simulink subsystem "Funcionamiento_motores"  (R2023b)
settings: Solver=VariableStepAuto  StartTime=0.0  StopTime=10.0  RelTol=1e-3
libraries: arduinolib x4
settings Model: Creator=Usuario_UMA  LastModifiedBy=juana

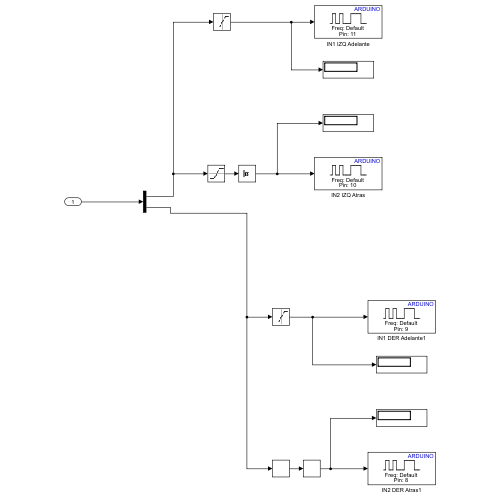
[thumbnail: Simulink's stored preview of the top-level diagram]
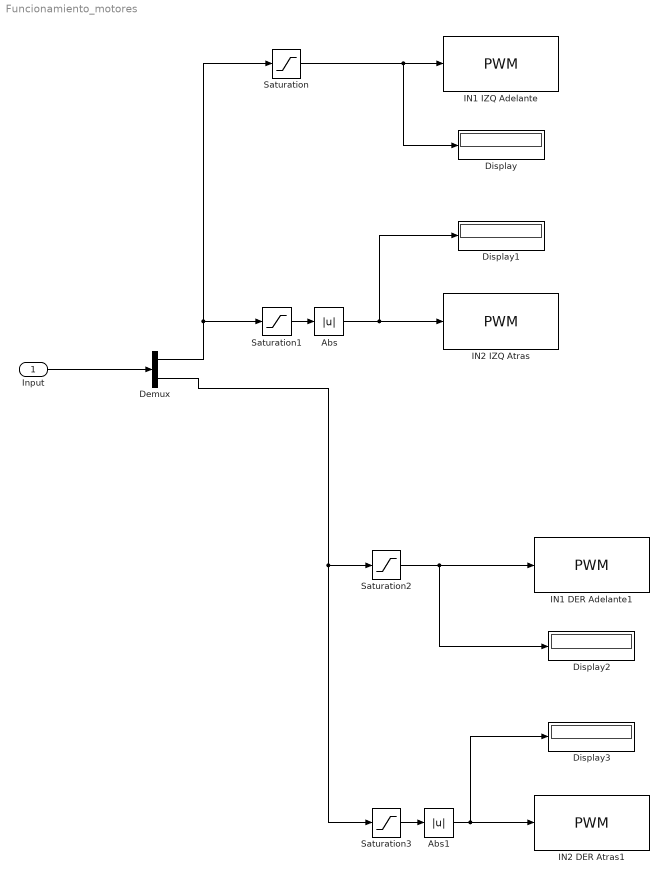
== system Funcionamiento_motores ==
  Input : Inport  OutMin=[-255]  OutMax=[255]
  Abs : Abs  SaturateOnIntegerOverflow=off
  Abs1 : Abs  SaturateOnIntegerOverflow=off
  Demux : Demux  Outputs=2
  Display{,1..3} (4 alike) : Display
  IN1 DER Adelante1 : arduinolib/PWM  pinNumber=9  frequencyType=Default  desiredFrequency=490.2  achievableFrequency=490.2
  IN1 IZQ Adelante : arduinolib/PWM  pinNumber=11  frequencyType=Default  desiredFrequency=490.2  achievableFrequency=490.2
  IN2 DER Atras1 : arduinolib/PWM  pinNumber=8  frequencyType=Default  desiredFrequency=490.2  achievableFrequency=490.2
  IN2 IZQ Atras : arduinolib/PWM  pinNumber=10  frequencyType=Default  desiredFrequency=490.2  achievableFrequency=490.2
  Saturation : Saturate  UpperLimit=255  LowerLimit=1
  Saturation1 : Saturate  UpperLimit=0  LowerLimit=-255
  Saturation2 : Saturate  UpperLimit=255  LowerLimit=1
  Saturation3 : Saturate  UpperLimit=0  LowerLimit=-255
  wires:
  Abs/1 -> Display1/1, IN2 IZQ Atras/1
  Input/1 -> Demux/1
  Demux/1 -> Saturation1/1, Saturation/1
  Abs1/1 -> Display3/1, IN2 DER Atras1/1
  Saturation/1 -> Display/1, IN1 IZQ Adelante/1
  Saturation1/1 -> Abs/1
  Saturation2/1 -> Display2/1, IN1 DER Adelante1/1
  Saturation3/1 -> Abs1/1
  Demux/2 -> Saturation3/1, Saturation2/1
